simulink model "SpringMassDamper"  (R2021a)
settings: Solver=VariableStepAuto  StartTime=0.0  StopTime=100  RelTol=1e-3
values from neighbouring files (symbols this model uses):
  d1 = 16    [Parameters.m]
  d2 = 10    [Parameters.m]
  F = 10    [Parameters.m]
  k1 = 10    [Parameters.m]
  k2 = 10    [Parameters.m]
  m1 = 20    [Parameters.m]
  m2 = 20    [Parameters.m]
settings Model: Creator=zurab  LastModifiedBy=zurab

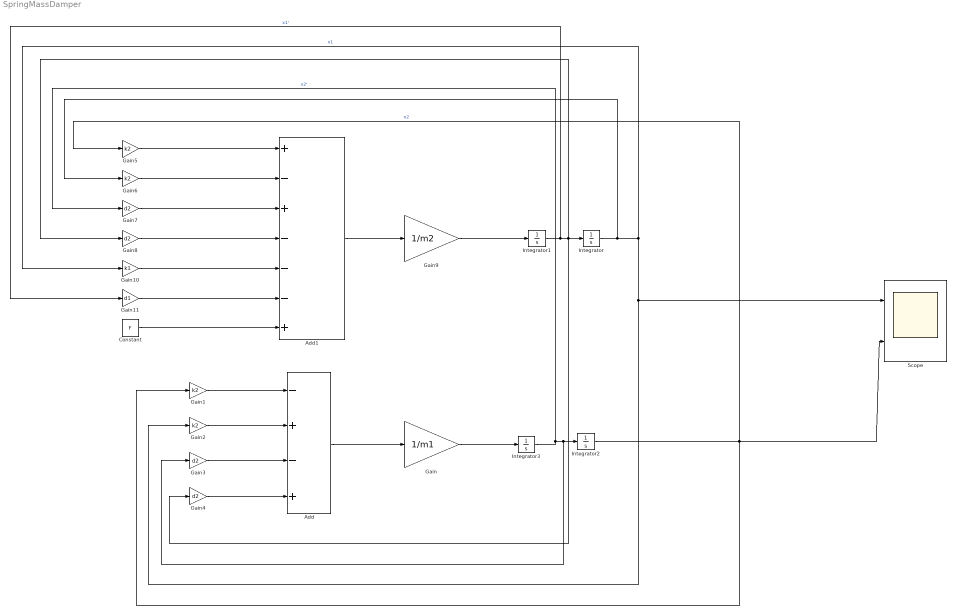
== system SpringMassDamper ==
  Add : Sum  Inputs=-+-+
  Add1 : Sum  Inputs=+-+---+
  Constant : Constant  Value=F
  Gain : Gain  Gain=1/m1
  Gain{1..2,5..6} (4 alike) : Gain  Gain=k2
  Gain10 : Gain  Gain=k1
  Gain11 : Gain  Gain=d1
  Gain{3..4,7..8} (4 alike) : Gain  Gain=d2
  Gain9 : Gain  Gain=1/m2
  Integrator{,1..3} (4 alike) : Integrator
  Scope : Scope  NumInputPorts=2
  wires:
  Integrator1/1 -> Gain11/1, Gain4/1, Gain8/1, Integrator/1  "x1'"
  Integrator3/1 -> Gain7/1, Gain3/1, Integrator2/1  "x2'"
  Integrator2/1 -> Gain5/1, Gain1/1, Scope/2  "x2"
  Add/1 -> Gain/1
  Gain/1 -> Integrator3/1
  Integrator/1 -> Gain2/1, Scope/1, Gain10/1, Gain6/1  "x1"
  Gain4/1 -> Add/4
  Gain3/1 -> Add/3
  Gain2/1 -> Add/2
  Gain1/1 -> Add/1
  Gain5/1 -> Add1/1
  Gain6/1 -> Add1/2
  Gain7/1 -> Add1/3
  Gain8/1 -> Add1/4
  Add1/1 -> Gain9/1
  Gain9/1 -> Integrator1/1
  Gain11/1 -> Add1/6
  Gain10/1 -> Add1/5
  Constant/1 -> Add1/7
